simulink model "chap8_5sim2015"  (R2015b)
settings: Solver=ode45  StartTime=0.0  StopTime=30  RelTol=1e-3
settings Model: Creator=zhr  LastModifiedBy=IT
settings DataIOCC: SaveFormat=Array
settings DebuggingCC: AllowSymbolicDim=on
settings HardwareCC: ProdBitPerPointer=32  ProdLargestAtomicFloat=None  ProdIntDivRoundTo=Undefined  ProdEndianess=Unspecified  ProdWordSize=32  ProdHWDeviceType=32-bit Generic
settings GRTTargetCC: GeneratePreprocessorConditionals=Disable all
settings ConfigComp: CovModelRefEnable=Off

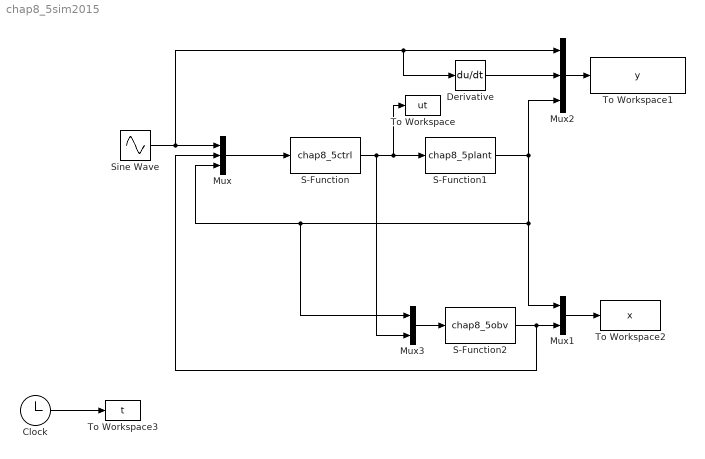
== system chap8_5sim2015 ==
  Clock : Clock
  Derivative : Derivative
  Mux : Mux  Inputs=3
  Mux1 : Mux  Inputs=2
  Mux2 : Mux  Inputs=3
  Mux3 : Mux  Inputs=2
  S-Function : S-Function  FunctionName=chap8_5ctrl  SFunctionDeploymentMode=off  EnableBusSupport=off
  S-Function1 : S-Function  FunctionName=chap8_5plant  SFunctionDeploymentMode=off  EnableBusSupport=off
  S-Function2 : S-Function  FunctionName=chap8_5obv  SFunctionDeploymentMode=off  EnableBusSupport=off
  Sine Wave : Sin  Frequency=2*pi/5  SampleTime=0
  To Workspace : ToWorkspace  VariableName=ut  SampleTime=-1
  To Workspace1 : ToWorkspace  VariableName=y  SampleTime=-1
  To Workspace2 : ToWorkspace  VariableName=x  SampleTime=-1
  To Workspace3 : ToWorkspace  VariableName=t  SampleTime=-1
  wires:
  Sine Wave/1 -> Derivative/1, Mux2/1, Mux/1
  Mux/1 -> S-Function/1
  S-Function/1 -> Mux3/2, To Workspace/1, S-Function1/1
  Mux1/1 -> To Workspace2/1
  S-Function1/1 -> Mux3/1, Mux/3, Mux1/1, Mux2/3
  Derivative/1 -> Mux2/2
  Mux3/1 -> S-Function2/1
  S-Function2/1 -> Mux/2, Mux1/2
  Mux2/1 -> To Workspace1/1
  Clock/1 -> To Workspace3/1
